simulink model "motorcontrol"  (R2022b)
settings: Solver=FixedStepAuto  StartTime=0.0  StopTime=inf  RelTol=1e-3
libraries: arduinolib x5, arduinosensorlib x1
settings Model: ExtModeTrigDuration=2  Creator=gevor  LastModifiedBy=gevor
settings OptimizationCC: EnhancedBackFolding=on  PassReuseOutputArgsThreshold=0  MaxStackSize=64  OptimizeBlockOrder=speed  DifferentSizesBufferReuse=on  OptimizationCustomize=off
settings DebuggingCC: ParameterTunabilityLossMsg=error  UnconnectedInputMsg=warning  UnconnectedOutputMsg=warning  UnconnectedLineMsg=warning
settings HardwareCC: ProdBitPerInt=16  ProdBitPerPointer=16  ProdBitPerSizeT=16  ProdBitPerPtrDiffT=16  ProdLargestAtomicFloat=None  ProdWordSize=8  ProdHWDeviceType=Atmel->AVR  UseEmbeddedCoderFeatures=off  UseSimulinkCoderFeatures=off
settings ModelReferenceCC: EnableRefExpFcnMdlSchedulingChecks=on
settings SFSimCC: MATLABDynamicMemAlloc=off
settings RTWCC: Description=Embedded Coder  SystemTargetFile=ert.tlc  HardwareBoard=Arduino Mega 2560  TLCOptions=-aInlineSetEventsForThisBaseRateFcn=TLC_FALSE -aSuppressMultiTaskScheduler=TLC_FALSE -aRateBasedStepFcn=1  TemplateMakefile=ert_default_tmf  Toolchain=Arduino AVR  DLArmComputeVersion=19.05
settings CodeAppCC: ForceParamTrailComments=on  OperatorAnnotations=on
settings ERTTargetCC: ERTCustomFileBanners=off  SupportContinuousTime=on  SupportNonInlinedSFcns=on  RemoveResetFunc=off  SupportVariableSizeSignals=on  ModelStepFunctionPrototypeControlCompliant=off  ExtModeStaticAllocSize=2048

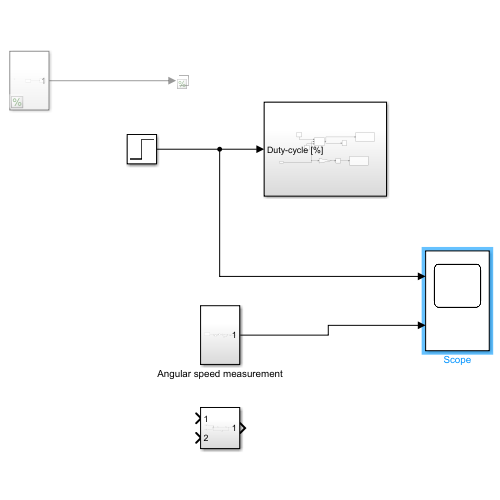
[thumbnail: Simulink's stored preview of the top-level diagram]
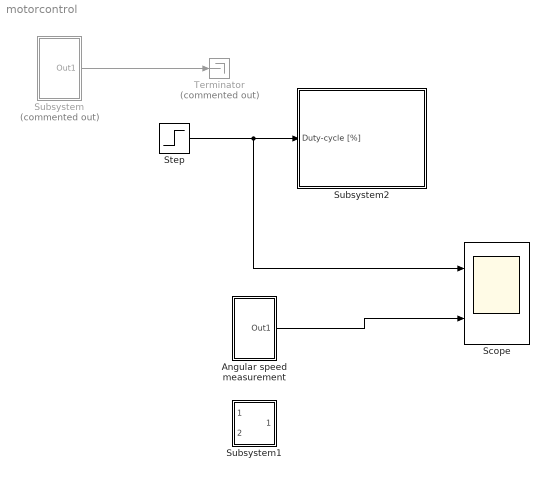
== system motorcontrol ==
  Angular speed measurement : Subsystem
  Scope : Scope  NumInputPorts=2
  Step : Step  Time=5  After=100  SampleTime=0
  Subsystem : Subsystem  Commented=on
  Subsystem1 : Subsystem
  Subsystem2 : Subsystem
  Terminator : Terminator  Commented=on
  wires:
  Subsystem/1(Out1) -> Terminator/1
  Angular speed measurement/1(Out1) -> Scope/2
  Step/1 -> Scope/1, Subsystem2/1(Duty-cycle [%])

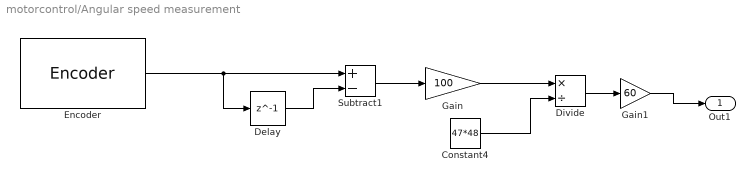
== system motorcontrol/Angular speed measurement ==
  Constant4 : Constant  Value=47*48
  Delay : Delay  DelayLength=1  SampleTime=0.01
  Divide : Product  Inputs=*/
  Encoder : arduinosensorlib/Encoder  InputA=20  InputB=21  Mode=No reset  SampleTime=.01
  Gain : Gain  Gain=100
  Gain1 : Gain  Gain=60
  Subtract1 : Sum  Inputs=+-
  Out1 : Outport
  wires:
  Gain1/1 -> Out1/1
  Encoder/1 -> Subtract1/1, Delay/1
  Gain/1 -> Divide/1
  Subtract1/1 -> Gain/1
  Constant4/1 -> Divide/2
  Divide/1 -> Gain1/1
  Delay/1 -> Subtract1/2

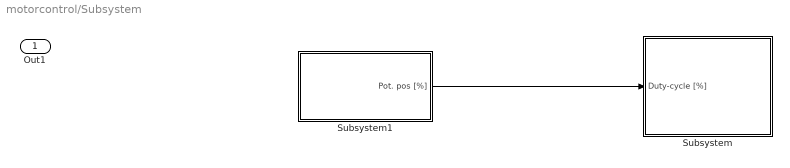
== system motorcontrol/Subsystem ==
  Subsystem : Subsystem
  Subsystem1 : Subsystem
  Out1 : Outport
  wires:
  Subsystem1/1(" Pot. pos [%]") -> Subsystem/1(Duty-cycle [%])

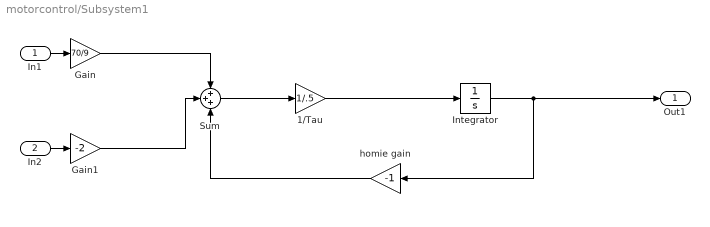
== system motorcontrol/Subsystem1 ==
  In1 : Inport
  In2 : Inport  Port=2
  1/Tau : Gain  Gain=1/.5
  Gain : Gain  Gain=70/9
  Gain1 : Gain  Gain=-2
  Integrator : Integrator
  Sum : Sum  Inputs=+++
  homie gain : Gain  Gain=-1
  Out1 : Outport
  wires:
  In1/1 -> Gain/1
  Sum/1 -> 1/Tau/1
  Gain/1 -> Sum/1
  homie gain/1 -> Sum/3
  Integrator/1 -> Out1/1, homie gain/1
  In2/1 -> Gain1/1
  Gain1/1 -> Sum/2
  1/Tau/1 -> Integrator/1

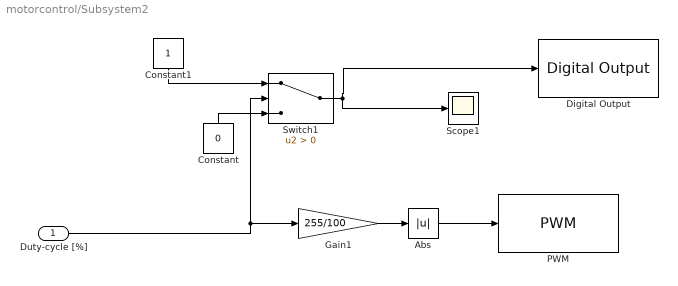
== system motorcontrol/Subsystem2 ==
  Duty-cycle [%] : Inport
  Abs : Abs  SaturateOnIntegerOverflow=off
  Constant : Constant  Value=0
  Constant1 : Constant
  Digital Output : arduinolib/Digital Output  pinNumber=13  Direction=output  blockPlatform=arduino
  Gain1 : Gain  Gain=255/100
  PWM : arduinolib/PWM  pinNumber=11  frequencyType=Default  desiredFrequency=490.2  achievableFrequency=490.2
  Scope1 : Scope
  Switch1 : Switch  Criteria=u2 > Threshold  SaturateOnIntegerOverflow=off  InputSameDT=off
  wires:
  Gain1/1 -> Abs/1
  Duty-cycle [%]/1 -> Switch1/2, Gain1/1
  Constant/1 -> Switch1/3
  Constant1/1 -> Switch1/1
  Switch1/1 -> Digital Output/1, Scope1/1
  Abs/1 -> PWM/1

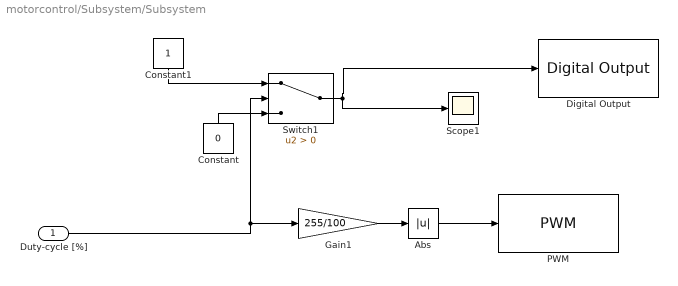
== system motorcontrol/Subsystem/Subsystem ==
  Duty-cycle [%] : Inport
  Abs : Abs  SaturateOnIntegerOverflow=off
  Constant : Constant  Value=0
  Constant1 : Constant
  Digital Output : arduinolib/Digital Output  pinNumber=13  Direction=output  blockPlatform=arduino
  Gain1 : Gain  Gain=255/100
  PWM : arduinolib/PWM  pinNumber=11  frequencyType=Default  desiredFrequency=490.2  achievableFrequency=490.2
  Scope1 : Scope
  Switch1 : Switch  Criteria=u2 > Threshold  SaturateOnIntegerOverflow=off  InputSameDT=off
  wires:
  Gain1/1 -> Abs/1
  Duty-cycle [%]/1 -> Switch1/2, Gain1/1
  Constant/1 -> Switch1/3
  Constant1/1 -> Switch1/1
  Switch1/1 -> Digital Output/1, Scope1/1
  Abs/1 -> PWM/1

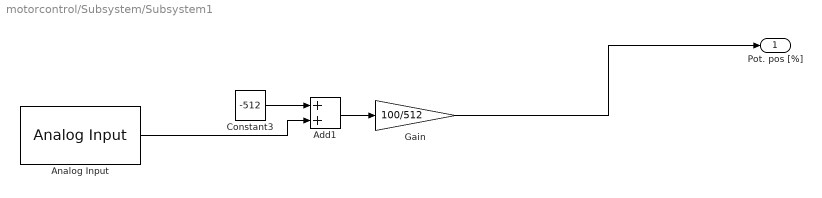
== system motorcontrol/Subsystem/Subsystem1 ==
  Add1 : Sum
  Analog Input : arduinolib/Analog Input  pinNumber=2  ReadResultsOnly=off  ConversionTriggerSource=Software  ExternalTriggerType=uint32( 0 )  OutputDataType=uint16  EnableConversionCompleteNotify=off  EnableOuputStatus=off  SampleTime=-1  blockPlatform=arduino
  Constant3 : Constant  Value=-512
  Gain : Gain  Gain=100/512
  " Pot. pos [%]" : Outport
  wires:
  Add1/1 -> Gain/1
  Constant3/1 -> Add1/1
  Analog Input/1 -> Add1/2
  Gain/1 -> " Pot. pos [%]"/1
